simulink model "Demo2022b"  (R2022b)
settings: Solver=FixedStepAuto  StartTime=0.0  StopTime=inf  RelTol=1e-3  EnableMultiTasking=on
settings Model: ExtModeTrigDuration=2  Creator=bryantboatright  LastModifiedBy=bryantboatright
settings SolverCC: AutoInsertRateTranBlk=on
settings OptimizationCC: EnhancedBackFolding=on  PassReuseOutputArgsAs=Individual arguments  ZeroExternalMemoryAtStartup=off  ZeroInternalMemoryAtStartup=off  MaxStackSize=64  OptimizeBlockOrder=speed  DifferentSizesBufferReuse=on  OptimizationCustomize=off  EfficientTunableParamExpr=on
settings DebuggingCC: ParameterTunabilityLossMsg=error
settings HardwareCC: ProdBitPerInt=16  ProdBitPerPointer=16  ProdBitPerSizeT=16  ProdBitPerPtrDiffT=16  ProdLargestAtomicFloat=None  ProdWordSize=8  ProdHWDeviceType=Atmel->AVR
settings RTWCC: Description=Embedded Coder  SystemTargetFile=ert.tlc  HardwareBoard=Arduino Uno  TLCOptions=-aInlineSetEventsForThisBaseRateFcn=TLC_FALSE -aSuppressMultiTaskScheduler=TLC_FALSE -aRateBasedStepFcn=1  TemplateMakefile=ert_default_tmf  Toolchain=Arduino AVR  BuildConfiguration=Faster Runs
settings CodeAppCC: ForceParamTrailComments=on  IgnoreCustomStorageClasses=off  OperatorAnnotations=on  SimulinkDataObjDesc=on  SFDataObjDesc=on  InsertBlockDesc=on
settings ERTTargetCC: TargetLangStandard=C99 (ISO)  SupportContinuousTime=on  SupportVariableSizeSignals=on  ExtModeTransport=3  ExtModeStaticAlloc=on  ExtModeAutomaticAllocSize=off  ExtModeStaticAllocSize=250  ExtModeMexFile=ext_xcp  ExtModeIntrfLevel=Level2 - Open

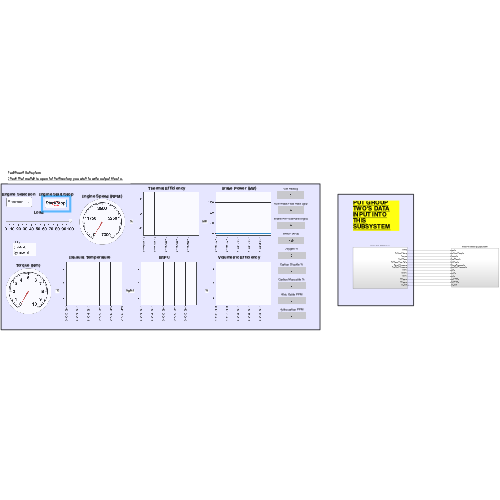
[thumbnail: Simulink's stored preview of the top-level diagram]
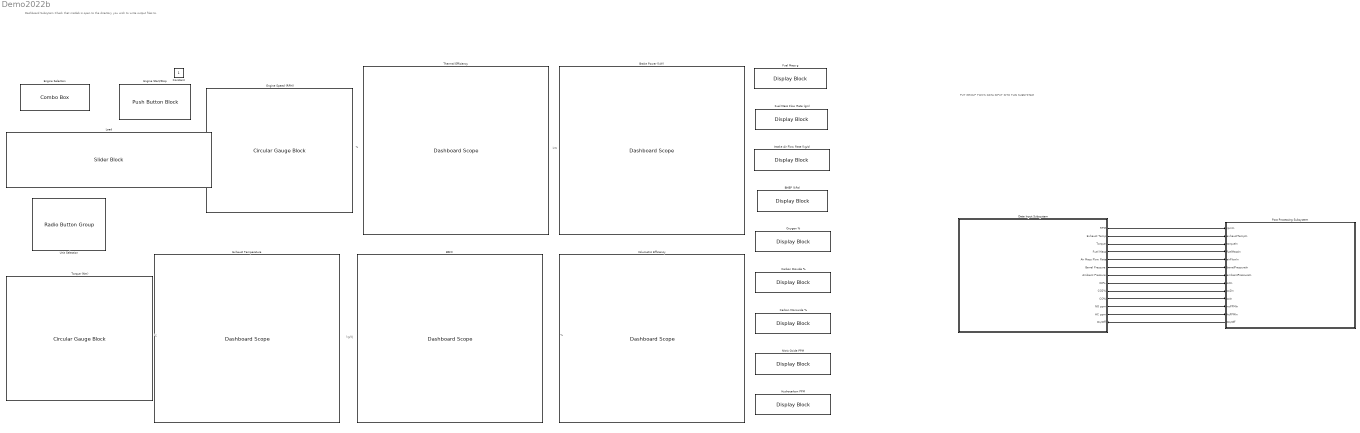
== system Demo2022b ==
  note: %
  note: Dashboard Subsytem
      |
      | Check that matlab is open to the directory you wish to write output files to.
  note: PUT GROUP TWO'S DATA INPUT INTO THIS SUBSYSTEM
  note: ˚C
  note: kg/kJ
  note: kW
  note: %
  BMEP (kPa) : DisplayBlock  LabelPosition=Hide  Transparency=1
  BSFC : DashboardScope  LegendPosition=Hide  UpdateMode=Scroll
  Brake Power (kW) : DashboardScope  LegendPosition=Hide  UpdateMode=Scroll
  Carbon Dioxide % : DisplayBlock  LabelPosition=Hide  Transparency=1
  Carbon Monoxide % : DisplayBlock  LabelPosition=Hide  Transparency=1
  Data Input Subsystem : Subsystem
      settings: PortSchema="{\"entries\":[{\"content\":{\"sides\":[{\"content\":{\"connectorIds\":[]},\"type\":\"ConnectorPlacement.EquallySpacedRectSide\",\"uuid\":\"3754a3e3-4518-42e3-a0cd-0eb816f7e60c\"},{\"content\":{\"connectorIds\":[\"Out1\",\"Out2\",\"Out3\",\"Out4\",\"Out5\",\"Out6\",\"Out7\",\"Out8\",\"Out9\",\"Out10\",\"Out11\",\"Out12\",\"In1\"],\"side\":\"RIGHT\"},\"type\":\"ConnectorPlacement.EquallySpacedRectSide\",\"uuid\":\"d3dfe676-b6e6-4c7f-98c7-8b108f201c07\"},{\"content\":{\"connectorIds\":[],\"side\":\"TOP\"},\"type\":\"ConnectorPlacement.EquallySpacedRectSide\",\"uuid\":\"2f91c8dd-0198-445b-930d-495fc8bcc849\"}]},\"type\":\"ConnectorPlacement.EquallySpacedConnector\",\"uuid\":\"520c6fba-fa44-47d2-96c9-29e04e3d0d93\"}],\"packageUris\":[\"http://schema.mathworks.com/mf0/Connector/R2020b\"],\"version\":\"1.0\"}"
  Engine Selection : ComboBox  LabelPosition=Hide  SelectedLabel=Yanmar
      settings: Values={{'Yanmar', 'Craftsman', 'John Deer', 'Chevy V6', 'Kohler', 'DuroMax'}, [1 2 3 4 5 6]}
  Engine Speed (RPM) : CircularGaugeBlock  LabelPosition=Hide  ScaleMax=7000  TickInterval=1750
  Engine Start/Stop : PushButtonBlock  ButtonText=Start/Stop  ButtonType=Latch  Icon=Engine  IconAlignment=Center  IconColor=On  OffValue=0.000000
  Exhaust Temperature : DashboardScope  LegendPosition=Hide  ScaleAtStop=off
  Fuel Mass Flow Rate (g/s) : DisplayBlock  LabelPosition=Hide  Transparency=1
  Fuel Mass g : DisplayBlock  LabelPosition=Hide  Transparency=1
  Hydrocarbon PPM : DisplayBlock  LabelPosition=Hide  Transparency=1
  Intake Air Flow Rate (kg/s) : DisplayBlock  LabelPosition=Hide  Transparency=1
  Load : SliderBlock  LabelPosition=Hide
  Nitric Oxide PPM : DisplayBlock  LabelPosition=Hide  Transparency=1
  Oxygen % : DisplayBlock  LabelPosition=Hide  Transparency=1
  Post Processing Subsystem : Subsystem
      settings: PortSchema="{\"entries\":[{\"content\":{\"sides\":[{\"content\":{\"connectorIds\":[\"In1\",\"In2\",\"In3\",\"In4\",\"In5\",\"In6\",\"In7\",\"In8\",\"In9\",\"In10\",\"In11\",\"In12\",\"Out1\"]},\"type\":\"ConnectorPlacement.EquallySpacedRectSide\",\"uuid\":\"2e8fbbbd-04f3-4cfb-b1cc-1db1e48dc879\"},{\"content\":{\"connectorIds\":[],\"side\":\"RIGHT\"},\"type\":\"ConnectorPlacement.EquallySpacedRectSide\",\"uuid\":\"1e86395c-1e99-406b-884b-92366c924b1f\"},{\"content\":{\"connectorIds\":[],\"side\":\"TOP\"},\"type\":\"ConnectorPlacement.EquallySpacedRectSide\",\"uuid\":\"23f1f2f5-9354-4dfe-ba19-9e9e16993f9b\"}]},\"type\":\"ConnectorPlacement.EquallySpacedConnector\",\"uuid\":\"bb08251b-5f96-4a99-a638-0e0833315a09\"}],\"packageUris\":[\"http://schema.mathworks.com/mf0/Connector/R2020b\"],\"version\":\"1.0\"}"
  Thermal Efficiency : DashboardScope  LegendPosition=Hide  UpdateMode=Scroll
  Torque (Nm) : CircularGaugeBlock  LabelPosition=Hide  ScaleMax=10  TickInterval=1
  Unit Selection : RadioButtonGroup  LabelPosition=Hide  SelectedLabel=Imperial  ButtonGroupName=Units
      settings: Values={{'Metric', 'Imperial'}, [0 1]}
  Volumetric Efficiency : DashboardScope  LegendPosition=Hide  UpdateMode=Scroll
  Constant : Constant  IOType=siggen
  wires:
  Data Input Subsystem/1(RPM) -> Post Processing Subsystem/1(rpmIn)
  Data Input Subsystem/2(Exhaust Temp) -> Post Processing Subsystem/2(exhaustTempIn)
  Data Input Subsystem/3(Torque) -> Post Processing Subsystem/3(torqueIn)
  Data Input Subsystem/4(Fuel Mass) -> Post Processing Subsystem/4(fuelMassIn)
  Data Input Subsystem/5(Air Mass Flow Rate) -> Post Processing Subsystem/5(airFlowIn)
  Data Input Subsystem/6(Barrel Pressure) -> Post Processing Subsystem/6(barrelPressureIn)
  Data Input Subsystem/7(Ambient Pressure) -> Post Processing Subsystem/7(ambientPressureIn)
  Data Input Subsystem/8(O2%) -> Post Processing Subsystem/8(o2In)
  Data Input Subsystem/9(CO2%) -> Post Processing Subsystem/9(co2In)
  Data Input Subsystem/10(CO%) -> Post Processing Subsystem/10(coIn)
  Data Input Subsystem/11(NO ppm) -> Post Processing Subsystem/11(noPPMIn)
  Data Input Subsystem/12(HC ppm) -> Post Processing Subsystem/12(hcPPMIn)
  Post Processing Subsystem/1(On/Off) -> Data Input Subsystem/1(On/Off)

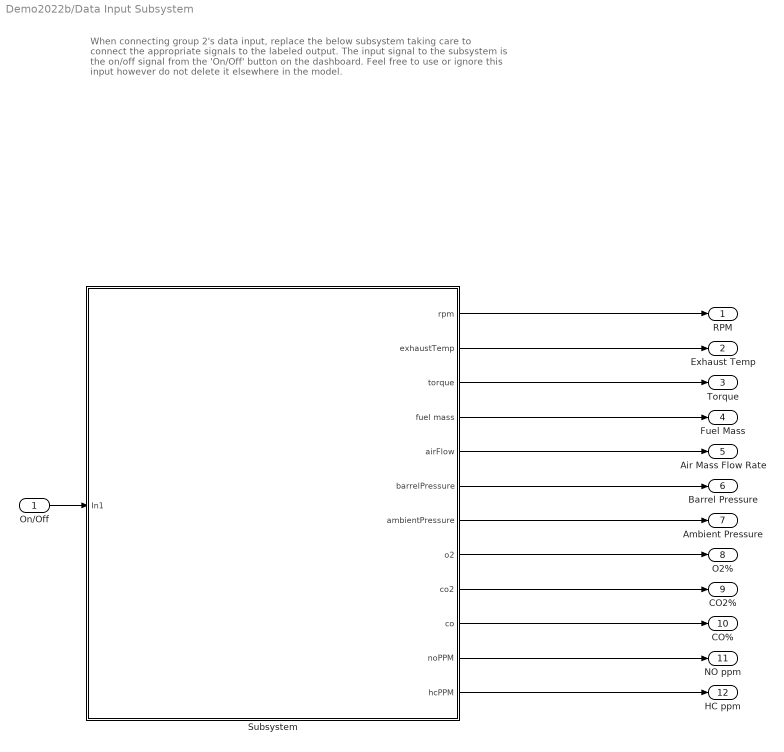
== system Demo2022b/Data Input Subsystem ==
  note: When connecting group 2's data input, replace the below subsystem taking care to connect the appropriate signals to the labeled output. The input signal to the subsystem is the on/off signal from the 'On/Off' button on the dashboard. Feel free to use or ignore this input however do not delete it elsewhere in the model.
  On/Off : Inport
  Subsystem : Subsystem
  RPM : Outport
  Exhaust Temp : Outport  Port=2
  Torque : Outport  Port=3
  Fuel Mass : Outport  Port=4
  Air Mass Flow Rate : Outport  Port=5
  Barrel Pressure : Outport  Port=6
  Ambient Pressure : Outport  Port=7
  O2% : Outport  Port=8
  CO2% : Outport  Port=9
  CO% : Outport  Port=10
  NO ppm : Outport  Port=11
  HC ppm : Outport  Port=12
  wires:
  Subsystem/1(rpm) -> RPM/1
  Subsystem/2(exhaustTemp) -> Exhaust Temp/1
  Subsystem/3(torque) -> Torque/1
  Subsystem/4(fuel mass) -> Fuel Mass/1
  Subsystem/5(airFlow) -> Air Mass Flow Rate/1
  Subsystem/6(barrelPressure) -> Barrel Pressure/1
  Subsystem/7(ambientPressure) -> Ambient Pressure/1
  Subsystem/8(o2) -> O2%/1
  Subsystem/9(co2) -> CO2%/1
  Subsystem/10(co) -> CO%/1
  Subsystem/11(noPPM) -> NO ppm/1
  Subsystem/12(hcPPM) -> HC ppm/1
  On/Off/1 -> Subsystem/1(In1)

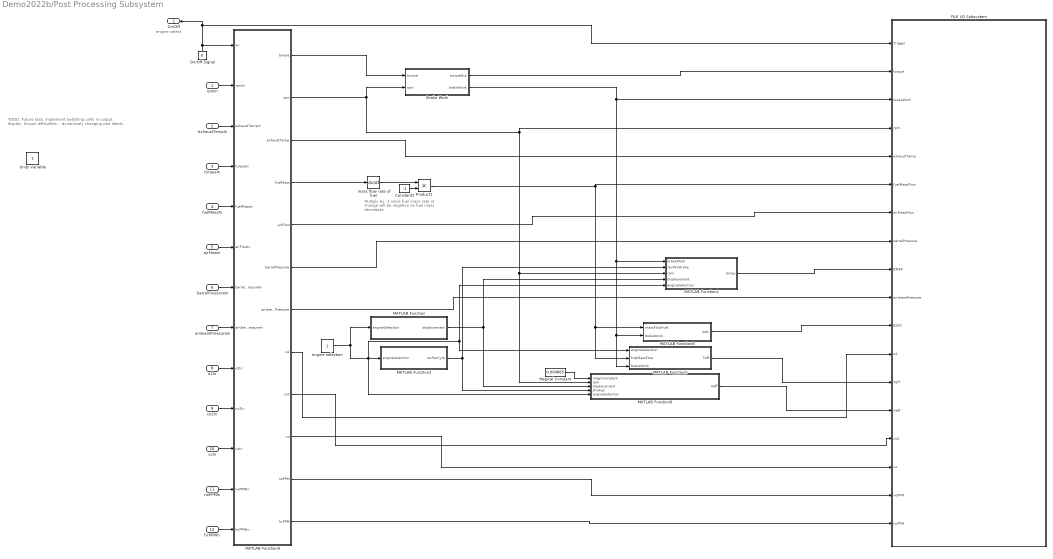
== system Demo2022b/Post Processing Subsystem ==
  note: Multiply by -1 since fuel mass rate of
      | change will be negative as fuel mass
      | decreases.
  note: TODO: Future task, implement switching units in output display.
      |
      | Known difficulties:
      | - dynamicaly changing plot labels.
  note: engine select
  rpmIn : Inport
  exhaustTempIn : Inport  Port=2
  torqueIn : Inport  Port=3
  fuelMassIn : Inport  Port=4
  airFlowIn : Inport  Port=5
  barrelPressureIn : Inport  Port=6
  ambientPressureIn : Inport  Port=7
  o2In : Inport  Port=8
  co2In : Inport  Port=9
  coIn : Inport  Port=10
  noPPMIn : Inport  Port=11
  hcPPMIn : Inport  Port=12
  Brake Work : MATLAB Function  TreatAsAtomicUnit=on
  Constant2 : Constant  Value=-1
  FILE I/O Subsystem : Subsystem
  MATLAB Function : MATLAB Function  TreatAsAtomicUnit=on
  MATLAB Function1 : MATLAB Function  TreatAsAtomicUnit=on
  MATLAB Function2 : MATLAB Function  TreatAsAtomicUnit=on
  MATLAB Function5 : MATLAB Function  TreatAsAtomicUnit=on
  MATLAB Function6 : MATLAB Function  TreatAsAtomicUnit=on
  MATLAB Function8 : MATLAB Function  TreatAsAtomicUnit=on
  MATLAB Function9 : MATLAB Function  TreatAsAtomicUnit=on
  Magical Constant : Constant  Value=0.004865
  On/Off Signal : Constant  Value=0
  Product1 : Product
  Units Variable : Constant
  engine selection : Constant
  mass flow rate of fuel : Derivative
  On/Off : Outport
  wires:
  Brake Work/2(brakeWork) -> MATLAB Function5/3(brakeWork), MATLAB Function8/2(brakeWork), MATLAB Function1/1(brakeWork), FILE I/O Subsystem/3(brakeWork)
  MATLAB Function2/1(revPerCyle) -> MATLAB Function1/2(revPerStroke), MATLAB Function6/4(strokes)
  Magical Constant/1 -> MATLAB Function6/1(magicConstant)
  MATLAB Function/1(displacement) -> MATLAB Function1/4(displacement), MATLAB Function6/3(displacement)
  hcPPMIn/1 -> MATLAB Function9/13(hcPPMIn)
  MATLAB Function9/4(fuelMass) -> mass flow rate of fuel/1
  MATLAB Function9/2(rpm) -> Brake Work/2(rpm), MATLAB Function6/2(rpm), MATLAB Function1/3(rpm), FILE I/O Subsystem/4(rpm)
  noPPMIn/1 -> MATLAB Function9/12(noPPMIn)
  MATLAB Function9/1(torque) -> Brake Work/1(torque)
  coIn/1 -> MATLAB Function9/11(coIn)
  engine selection/1 -> MATLAB Function/1(engineSelection), MATLAB Function6/5(engineSelection), MATLAB Function1/5(engineSelection), MATLAB Function5/1(engineSelection), MATLAB Function2/1(engineSelection)
  co2In/1 -> MATLAB Function9/10(co2In)
  exhaustTempIn/1 -> MATLAB Function9/3(exhaustTempIn)
  ambientPressureIn/1 -> MATLAB Function9/8(ambientPressureIn)
  rpmIn/1 -> MATLAB Function9/2(rpmIn)
  fuelMassIn/1 -> MATLAB Function9/5(fuelMassIn)
  o2In/1 -> MATLAB Function9/9(o2In)
  barrelPressureIn/1 -> MATLAB Function9/7(barrelPressureIn)
  torqueIn/1 -> MATLAB Function9/4(torqueIn)
  airFlowIn/1 -> MATLAB Function9/6(airFlowIn)
  On/Off Signal/1 -> On/Off/1, FILE I/O Subsystem/1(Trigger), MATLAB Function9/1(on)
  Constant2/1 -> Product1/2
  Product1/1 -> MATLAB Function5/2(fuelMassFlow), MATLAB Function8/1(massFlowFuel), FILE I/O Subsystem/6(fuelMassFlow)
  mass flow rate of fuel/1 -> Product1/1
  Brake Work/1(torqueOut) -> FILE I/O Subsystem/2(torque)
  MATLAB Function9/3(exhaustTemp) -> FILE I/O Subsystem/5(exhaustTemp)
  MATLAB Function9/5(airFlow) -> FILE I/O Subsystem/7(airMassFlow)
  MATLAB Function9/6(barrelPressure) -> FILE I/O Subsystem/8(barrelPressure)
  MATLAB Function1/1(bmep) -> FILE I/O Subsystem/9(BMEP)
  MATLAB Function9/7(ambientPressure) -> FILE I/O Subsystem/10(ambientPressure)
  MATLAB Function8/1(bsfc) -> FILE I/O Subsystem/11(BSFC)
  MATLAB Function9/8(o2) -> FILE I/O Subsystem/12(o2)
  MATLAB Function5/1(Teff) -> FILE I/O Subsystem/13(Teff)
  MATLAB Function6/1(Veff) -> FILE I/O Subsystem/14(Veff)
  MATLAB Function9/9(co2) -> FILE I/O Subsystem/15(co2)
  MATLAB Function9/10(co) -> FILE I/O Subsystem/16(co)
  MATLAB Function9/11(noPPM) -> FILE I/O Subsystem/17(noPPM)
  MATLAB Function9/12(hcPPM) -> FILE I/O Subsystem/18(hcPPM)

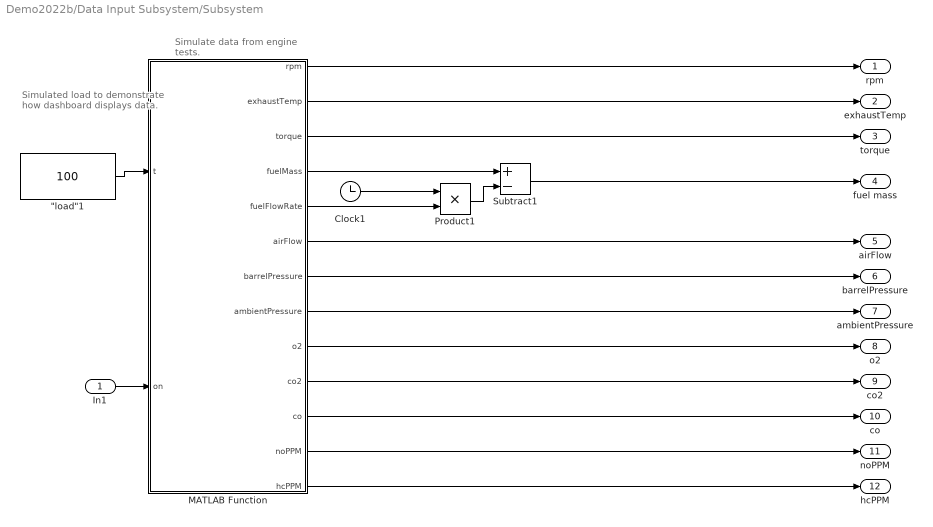
== system Demo2022b/Data Input Subsystem/Subsystem ==
  note: Simulated load to demonstrate how
      | dashboard displays data.
  note: Simulate data from engine
      | tests.
  In1 : Inport
  "\"load\"1" : Constant  Value=100
  Clock1 : Clock
  MATLAB Function : MATLAB Function  TreatAsAtomicUnit=on
  Product1 : Product
  Subtract1 : Sum  Inputs=+-
  rpm : Outport
  exhaustTemp : Outport  Port=2
  torque : Outport  Port=3
  fuel mass : Outport  Port=4
  airFlow : Outport  Port=5
  barrelPressure : Outport  Port=6
  ambientPressure : Outport  Port=7
  o2 : Outport  Port=8
  co2 : Outport  Port=9
  co : Outport  Port=10
  noPPM : Outport  Port=11
  hcPPM : Outport  Port=12
  wires:
  MATLAB Function/3(torque) -> torque/1
  MATLAB Function/13(hcPPM) -> hcPPM/1
  MATLAB Function/6(airFlow) -> airFlow/1
  MATLAB Function/5(fuelFlowRate) -> Product1/2
  MATLAB Function/12(noPPM) -> noPPM/1
  MATLAB Function/7(barrelPressure) -> barrelPressure/1
  MATLAB Function/8(ambientPressure) -> ambientPressure/1
  In1/1 -> MATLAB Function/2(on)
  MATLAB Function/9(o2) -> o2/1
  "\"load\"1"/1 -> MATLAB Function/1(t)
  MATLAB Function/4(fuelMass) -> Subtract1/1
  MATLAB Function/11(co) -> co/1
  MATLAB Function/10(co2) -> co2/1
  Product1/1 -> Subtract1/2
  Clock1/1 -> Product1/1
  Subtract1/1 -> fuel mass/1
  MATLAB Function/2(exhaustTemp) -> exhaustTemp/1
  MATLAB Function/1(rpm) -> rpm/1

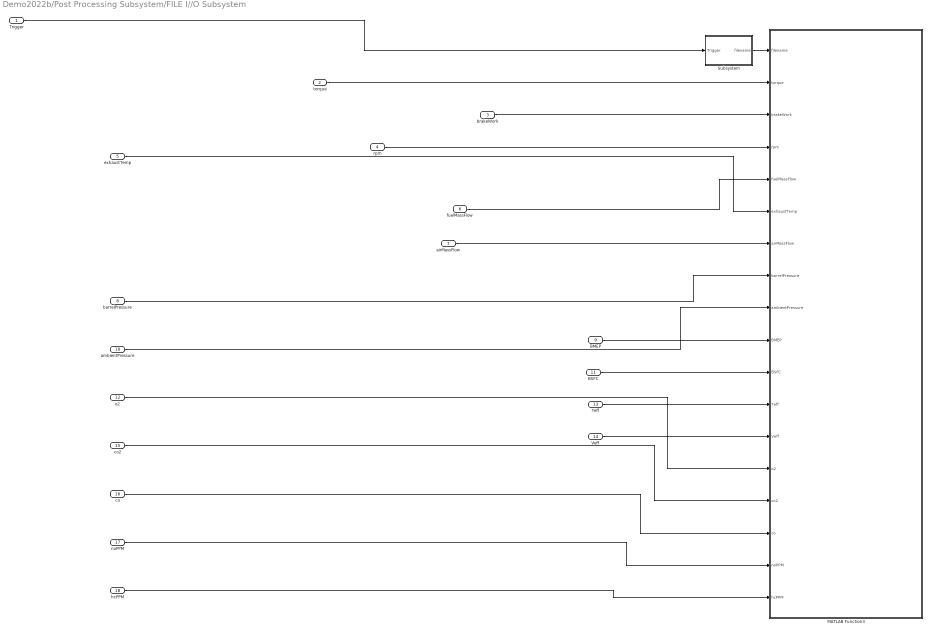
== system Demo2022b/Post Processing Subsystem/FILE I//O Subsystem ==
  Trigger : Inport
  torque : Inport  Port=2
  brakeWork : Inport  Port=3
  rpm : Inport  Port=4
  exhaustTemp : Inport  Port=5
  fuelMassFlow : Inport  Port=6
  airMassFlow : Inport  Port=7
  barrelPressure : Inport  Port=8
  BMEP : Inport  Port=9
  ambientPressure : Inport  Port=10
  BSFC : Inport  Port=11
  o2 : Inport  Port=12
  Teff : Inport  Port=13
  Veff : Inport  Port=14
  co2 : Inport  Port=15
  co : Inport  Port=16
  noPPM : Inport  Port=17
  hcPPM : Inport  Port=18
  MATLAB Function3 : MATLAB Function  TreatAsAtomicUnit=on
  Subsystem : Subsystem
  wires:
  noPPM/1 -> MATLAB Function3/17(noPPM)
  brakeWork/1 -> MATLAB Function3/3(brakeWork)
  exhaustTemp/1 -> MATLAB Function3/6(exhaustTemp)
  Veff/1 -> MATLAB Function3/13(Veff)
  barrelPressure/1 -> MATLAB Function3/8(barrelPressure)
  fuelMassFlow/1 -> MATLAB Function3/5(fuelMassFlow)
  o2/1 -> MATLAB Function3/14(o2)
  torque/1 -> MATLAB Function3/2(torque)
  Trigger/1 -> Subsystem/1(Trigger)
  Teff/1 -> MATLAB Function3/12(Teff)
  ambientPressure/1 -> MATLAB Function3/9(ambientPressure)
  BMEP/1 -> MATLAB Function3/10(BMEP)
  hcPPM/1 -> MATLAB Function3/18(hcPPM)
  airMassFlow/1 -> MATLAB Function3/7(airMassFlow)
  co/1 -> MATLAB Function3/16(co)
  Subsystem/1(filename) -> MATLAB Function3/1(filename)
  rpm/1 -> MATLAB Function3/4(rpm)
  co2/1 -> MATLAB Function3/15(co2)
  BSFC/1 -> MATLAB Function3/11(BSFC)

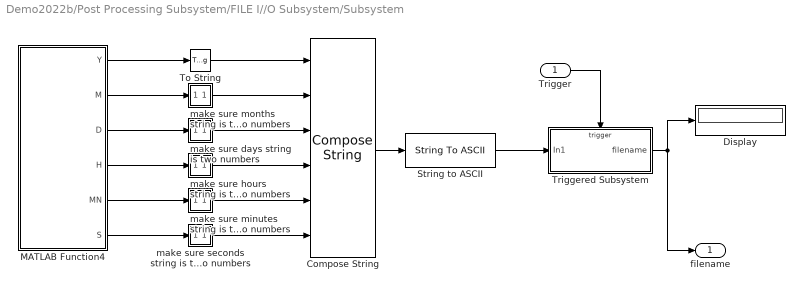
== system Demo2022b/Post Processing Subsystem/FILE I//O Subsystem/Subsystem ==
  Trigger : Inport
  Compose String : ComposeString  Format="\"%s-%s-%s--%s-%s-%s-output.csv\""
  Display : Display
  MATLAB Function4 : MATLAB Function  TreatAsAtomicUnit=on  SystemSampleTime=200
  String to ASCII : StringToASCII
  To String : ToString
  Triggered Subsystem : Subsystem  TreatAsAtomicUnit=on
  make sure days string is two numbers : Subsystem
  make sure hours string is two numbers : Subsystem
  make sure minutes string is two numbers : Subsystem
  make sure months string is two numbers : Subsystem
  make sure seconds string is two numbers : Subsystem
  filename : Outport
  wires:
  make sure months string is two numbers/1(Out1) -> Compose String/2
  To String/1 -> Compose String/1
  MATLAB Function4/6(S) -> make sure seconds string is two numbers/1(In1)
  Compose String/1 -> String to ASCII/1
  MATLAB Function4/5(MN) -> make sure minutes string is two numbers/1(In1)
  make sure days string is two numbers/1(Out1) -> Compose String/3
  make sure minutes string is two numbers/1(Out1) -> Compose String/5
  MATLAB Function4/4(H) -> make sure hours string is two numbers/1(In1)
  make sure hours string is two numbers/1(Out1) -> Compose String/4
  Trigger/1 -> Triggered Subsystem/Trigger
  MATLAB Function4/2(M) -> make sure months string is two numbers/1(In1)
  Triggered Subsystem/1(filename) -> filename/1, Display/1
  MATLAB Function4/3(D) -> make sure days string is two numbers/1(In1)
  MATLAB Function4/1(Y) -> To String/1
  make sure seconds string is two numbers/1(Out1) -> Compose String/6
  String to ASCII/1 -> Triggered Subsystem/1(In1)

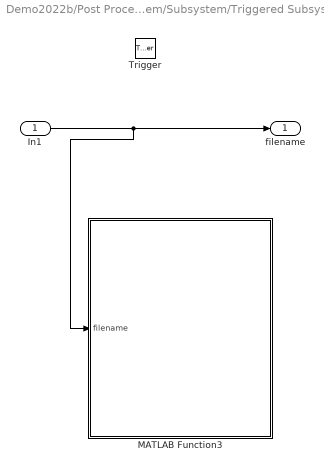
== system Demo2022b/Post Processing Subsystem/FILE I//O Subsystem/Subsystem/Triggered Subsystem ==
  In1 : Inport
  Trigger : TriggerPort  VariantControl=(inherit)
  MATLAB Function3 : MATLAB Function  TreatAsAtomicUnit=on
  filename : Outport
  wires:
  In1/1 -> MATLAB Function3/1(filename), filename/1

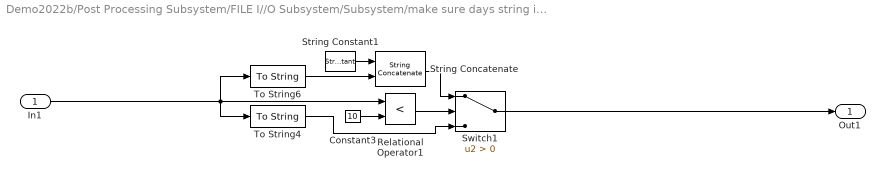
== system Demo2022b/Post Processing Subsystem/FILE I//O Subsystem/Subsystem/make sure days string is two numbers ==
  In1 : Inport
  Constant3 : Constant  Value=10  VectorParams1D=off  OutDataTypeStr=int8
  Relational Operator1 : RelationalOperator  Operator=<  OutDataTypeStr=boolean  RndMeth=Simplest  InputSameDT=off
  String Concatenate : StringConcatenate
  String Constant1 : StringConstant  String="\"0\""
  Switch1 : Switch  Criteria=u2 > Threshold  SaturateOnIntegerOverflow=off  InputSameDT=off
  To String4 : ToString
  To String6 : ToString
  Out1 : Outport
  wires:
  Constant3/1 -> Relational Operator1/2
  Relational Operator1/1 -> Switch1/2
  To String4/1 -> Switch1/3
  To String6/1 -> String Concatenate/2
  String Constant1/1 -> String Concatenate/1
  String Concatenate/1 -> Switch1/1
  In1/1 -> Relational Operator1/1, To String4/1, To String6/1
  Switch1/1 -> Out1/1

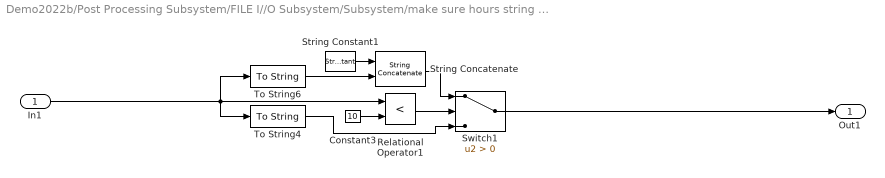
== system Demo2022b/Post Processing Subsystem/FILE I//O Subsystem/Subsystem/make sure hours string is two numbers ==
  In1 : Inport
  Constant3 : Constant  Value=10  VectorParams1D=off  OutDataTypeStr=int8
  Relational Operator1 : RelationalOperator  Operator=<  OutDataTypeStr=boolean  RndMeth=Simplest  InputSameDT=off
  String Concatenate : StringConcatenate
  String Constant1 : StringConstant  String="\"0\""
  Switch1 : Switch  Criteria=u2 > Threshold  SaturateOnIntegerOverflow=off  InputSameDT=off
  To String4 : ToString
  To String6 : ToString
  Out1 : Outport
  wires:
  Switch1/1 -> Out1/1
  In1/1 -> To String6/1, To String4/1, Relational Operator1/1
  String Concatenate/1 -> Switch1/1
  String Constant1/1 -> String Concatenate/1
  To String6/1 -> String Concatenate/2
  To String4/1 -> Switch1/3
  Relational Operator1/1 -> Switch1/2
  Constant3/1 -> Relational Operator1/2

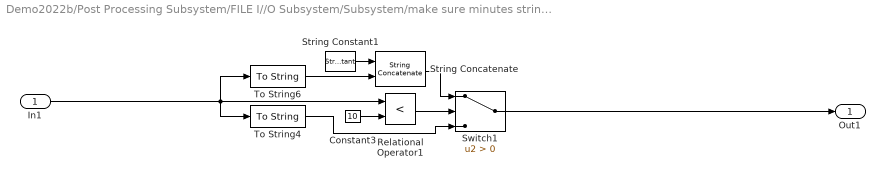
== system Demo2022b/Post Processing Subsystem/FILE I//O Subsystem/Subsystem/make sure minutes string is two numbers ==
  In1 : Inport
  Constant3 : Constant  Value=10  VectorParams1D=off  OutDataTypeStr=int8
  Relational Operator1 : RelationalOperator  Operator=<  OutDataTypeStr=boolean  RndMeth=Simplest  InputSameDT=off
  String Concatenate : StringConcatenate
  String Constant1 : StringConstant  String="\"0\""
  Switch1 : Switch  Criteria=u2 > Threshold  SaturateOnIntegerOverflow=off  InputSameDT=off
  To String4 : ToString
  To String6 : ToString
  Out1 : Outport
  wires:
  Constant3/1 -> Relational Operator1/2
  Relational Operator1/1 -> Switch1/2
  To String4/1 -> Switch1/3
  To String6/1 -> String Concatenate/2
  String Constant1/1 -> String Concatenate/1
  String Concatenate/1 -> Switch1/1
  In1/1 -> Relational Operator1/1, To String4/1, To String6/1
  Switch1/1 -> Out1/1

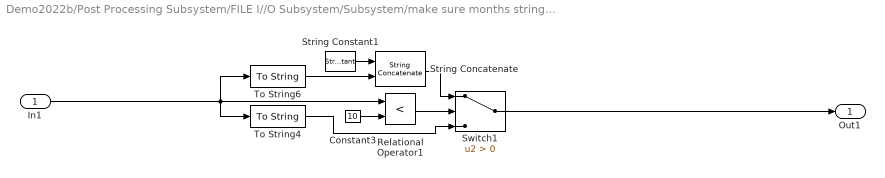
== system Demo2022b/Post Processing Subsystem/FILE I//O Subsystem/Subsystem/make sure months string is two numbers ==
  In1 : Inport
  Constant3 : Constant  Value=10  VectorParams1D=off  OutDataTypeStr=int8
  Relational Operator1 : RelationalOperator  Operator=<  OutDataTypeStr=boolean  RndMeth=Simplest  InputSameDT=off
  String Concatenate : StringConcatenate
  String Constant1 : StringConstant  String="\"0\""
  Switch1 : Switch  Criteria=u2 > Threshold  SaturateOnIntegerOverflow=off  InputSameDT=off
  To String4 : ToString
  To String6 : ToString
  Out1 : Outport
  wires:
  Switch1/1 -> Out1/1
  In1/1 -> To String6/1, To String4/1, Relational Operator1/1
  String Concatenate/1 -> Switch1/1
  String Constant1/1 -> String Concatenate/1
  To String6/1 -> String Concatenate/2
  To String4/1 -> Switch1/3
  Relational Operator1/1 -> Switch1/2
  Constant3/1 -> Relational Operator1/2

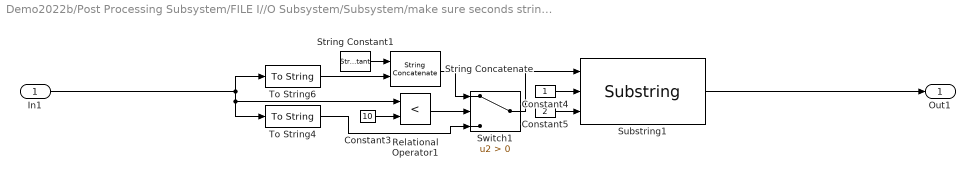
== system Demo2022b/Post Processing Subsystem/FILE I//O Subsystem/Subsystem/make sure seconds string is two numbers ==
  In1 : Inport
  Constant3 : Constant  Value=10  VectorParams1D=off  OutDataTypeStr=int8
  Constant4 : Constant  VectorParams1D=off  OutDataTypeStr=int8
  Constant5 : Constant  Value=2  VectorParams1D=off  OutDataTypeStr=uint8
  Relational Operator1 : RelationalOperator  Operator=<  OutDataTypeStr=boolean  RndMeth=Simplest  InputSameDT=off
  String Concatenate : StringConcatenate
  String Constant1 : StringConstant  String="\"0\""
  Substring1 : Substring
  Switch1 : Switch  Criteria=u2 > Threshold  SaturateOnIntegerOverflow=off  InputSameDT=off
  To String4 : ToString
  To String6 : ToString
  Out1 : Outport
  wires:
  Substring1/1 -> Out1/1
  To String4/1 -> Switch1/3
  Switch1/1 -> Substring1/1
  Constant3/1 -> Relational Operator1/2
  Constant5/1 -> Substring1/3
  In1/1 -> Relational Operator1/1, To String4/1, To String6/1
  Constant4/1 -> Substring1/2
  Relational Operator1/1 -> Switch1/2
  To String6/1 -> String Concatenate/2
  String Constant1/1 -> String Concatenate/1
  String Concatenate/1 -> Switch1/1

== matlab function Demo2022b/Post Processing Subsystem/MATLAB Function6 ==
  data: magicConstant input; Veff output; rpm input; displacement input; strokes input; engineSelection input
% Calculate Volumetric Efficiency
function Veff = calcVolumetricEfficiency(magicConstant, rpm, displacement, strokes, engineSelection)
if(engineSelection == 1 || engineSelection == 2 || engineSelection == 5 || engineSelection == 6)
    Veff = ((strokes * magicConstant) / (1.205 * displacement * (rpm / 60)));
elseif (engineSelection == 3)
    Veff = ((strokes * magicConstant) / (1.205 * (displacement * 4) * (rpm / 60)));
else
    Veff = ((strokes * magicConstant) / (1.205 * (displacement * 6) * (rpm / 60)));
end

== matlab function Demo2022b/Post Processing Subsystem/FILE I//O Subsystem/Subsystem/MATLAB Function4 ==
  data: Y output; M output; D output; H output; MN output; S output
function [Y, M, D, H, MN, S] = dateGenerator()
   Y = 0;
   M = 0;
   D = 0;
   H = 0;
   MN = 0;
   S = 0;
   [Y, M, D, H, MN, S] = datevec(datetime("now"));
end

== matlab function Demo2022b/Post Processing Subsystem/MATLAB Function8 ==
  data: massFlowFuel input; bsfc output; brakeWork input
% calculate BSFC based on fuel mass flow rate (kg/s) and Brake Work (Nm).
function bsfc = calcBSFC(massFlowFuel,brakeWork)

bsfc = massFlowFuel./brakeWork;

== matlab function Demo2022b/Post Processing Subsystem/MATLAB Function9 ==
  data: torque output; rpm output; exhaustTemp output; fuelMass output; airFlow output; barrelPressure output; ambientPressure output; on input; o2 output; co2 output; co output; noPPM output; hcPPM output; rpmIn input; exhaustTempIn input; torqueIn input; fuelMassIn input; airFlowIn input; barrelPressureIn input; ambientPressureIn input; o2In input; co2In input; coIn input; noPPMIn input; hcPPMIn input
% function to take input of 
%
% returns:
%
%   rpm: engine     speed rev per minute
%   exhaustTemp:    exhaust temperature in celsius
%   torque:         torque in Newton-meters
%   torqueMeasured: boolean - true if torque is measured, false if not
%   volts:          voltage
%   amps:           current
%   fuelMass:       mass of fuel container at current time.
%   

function [ torque,rpm,exhaustTemp,fuelMass,airFlow,barrelPressure,ambientPressure,...
    o2,co2,co,noPPM,hcPPM ] = fcn(on,rpmIn,exhaustTempIn,torqueIn,fuelMassIn,...
    airFlowIn,barrelPressureIn,ambientPressureIn,o2In,co2In,coIn,noPPMIn,hcPPMIn)
if(on == 1)
    rpm = rpmIn;
    exhaustTemp = exhaustTempIn;
    torque = torqueIn;
    fuelMass = fuelMassIn;
    airFlow = airFlowIn;
    barrelPressure = barrelPressureIn;
    ambientPressure = ambientPressureIn;
    o2 = o2In;
    co2 = co2In;
    co = coIn;
    noPPM = noPPMIn;
    hcPPM = hcPPMIn;
else
    rpm = 0;
    exhaustTemp = 0;
    torque = 0;
    fuelMass = 0;
    airFlow = 0;
    barrelPressure = 0;
    ambientPressure = 0;
    o2 = 0;
    co2 = 0;
    co = 0;
    noPPM = 0;
    hcPPM = 0;
end

== matlab function Demo2022b/Post Processing Subsystem/FILE I//O Subsystem/MATLAB Function3 ==
  data: filename input; torque input; brakeWork input; rpm input; fuelMassFlow input; exhaustTemp input; airMassFlow input; barrelPressure input; ambientPressure input; BMEP input; BSFC input; Teff input; Veff input; o2 input; co2 input; co input; noPPM input; hcPPM input
% log file generation - currently overwrites each run
% \r\n used for windows line termination style CRLF - switch to just \n if
% using unix like system
function fileOutput(filename,torque,brakeWork,rpm,fuelMassFlow,exhaustTemp,airMassFlow,barrelPressure,ambientPressure,BMEP,BSFC,Teff,Veff,o2,co2,co,noPPM,hcPPM)
if ([0 0] ~= size(double(char(filename))))
    file = fopen(char(filename),'a');
    if (0 > file)
        return
    end

    fprintf(file,'%.3f,%.3f,%.3f,%.3f,%.3f,%.3f,%.3f,%.3f,%.3f,%.3f,%.3f,%.3f,%.3f,%.3f,%.3f,%.3f,%.3f\r\n', ...
        torque,brakeWork,rpm,fuelMassFlow,exhaustTemp,airMassFlow,barrelPressure,ambientPressure,BMEP,BSFC,Teff,Veff,o2,co2,co,noPPM,hcPPM);
    fclose(file);
end

== matlab function Demo2022b/Post Processing Subsystem/FILE I//O Subsystem/Subsystem/Triggered Subsystem/MATLAB Function3 ==
  data: filename input
% log file generation - currently overwrites each run
% \r\n used for windows line termination style CRLF - switch to just \n if
% using unix like system
function fileOutput(filename)

if (0 ~= size(double(char(filename))))
    file = fopen(char(filename),'a');
    if (0 > file)
        return
    end

    fprintf(file,['torque,brakeWork,rpm,fuel mass flow,exhaust temperature,air mass flow..' ...
        ',barrel pressure,ambient pressure,BMEP,BSFC,thermal efficiency,...' ...
        'volumetric efficiency,o2,co2,co,no PPM,hc PPM\r\n']);
    fclose(file);
end

== matlab function Demo2022b/Post Processing Subsystem/MATLAB Function1 ==
  data: brakeWork input; bmep output; revPerStroke input; rpm input; displacement input; engineSelection input
% Calculate Brake Mean Effective Pressure (kPa).
function bmep = calcBMEP(brakeWork, revPerStroke, rpm,  displacement, engineSelection)
if(engineSelection == 1 || engineSelection == 2 || engineSelection == 5 || engineSelection ==6)
    bmep = ((brakeWork/((rpm/60)/revPerStroke))/displacement)/1000;
elseif(engineSelection==3)
     bmep = ((brakeWork/((rpm/60)/revPerStroke))/(displacement*4))/1000;
else
     bmep = ((brakeWork/((rpm/60)/revPerStroke))/(displacement*6))/1000;
end

== matlab function Demo2022b/Post Processing Subsystem/MATLAB Function ==
  data: displacement output; engineSelection input
% Set engine displacement (m^3) based on dropdown menu choice from dashboard
function displacement = pickDisplacement(engineSelection)
data = [0.000296 0.000196 0.000475 000.0004667 0.000429 0.000225];

displacement = data(1,engineSelection);

== matlab function Demo2022b/Post Processing Subsystem/MATLAB Function2 ==
  data: revPerCyle output; engineSelection input
% Set revolutions per cycle ( 1 for 2-stroke, 2 for 4-stroke ) based on
% engine selection from drop down menu on dashboard.
function revPerCyle = pickRevPerStroke(engineSelection)
data = [4 4 4 4 4 4];
revPerCyle = data(1,engineSelection);

== matlab function Demo2022b/Post Processing Subsystem/Brake Work ==
  data: torque input; torqueOut output; rpm input; brakeWork output
% Calculate Brake Work (kW/s) based on Engine Speed (rpm) and Torque (Nm)
function [torqueOut,brakeWork] = calcBrakeWork(torque,rpm)
brakeWork = 2 * pi * (rpm/60.0) * torque;

% Using diff name to reduce confusions. Torque only used in this function
% so to clean up lines was brought into this function.
torqueOut = torque;

== matlab function Demo2022b/Data Input Subsystem/Subsystem/MATLAB Function ==
  data: t input; rpm output; on input; exhaustTemp output; torque output; fuelMass output; fuelFlowRate output; airFlow output; barrelPressure output; ambientPressure output; o2 output; co2 output; co output; noPPM output; hcPPM output
function [ rpm,exhaustTemp,torque,fuelMass,fuelFlowRate,airFlow,barrelPressure,ambientPressure,...
    o2,co2,co,noPPM,hcPPM ] = fcn(t,on)
if (on)
    data = (1 + t / 100.0) * [ 2000 125 2.258 2000.0 0.004 0.94 3.4 16.5 0.003 35 59 0.004 ];
    rpm = data(1);
    exhaustTemp = data(2);
    torque = data(3);
    fuelMass = data(4);
    airFlow = data(5);
    barrelPressure = data(6);
    ambientPressure = 29;
    o2 = data(7);
    co2 = data(8);
    co = data(9);
    noPPM = data(10);
    hcPPM = data(11);
    fuelFlowRate = data(12);
else
    rpm = 0;
    exhaustTemp = 0;
    torque = 0;
    fuelMass = 0;
    airFlow = 0;
    barrelPressure = 0;
    ambientPressure = 0;
    o2 = 0;
    co2 = 0;
    co = 0;
    noPPM = 0;
    hcPPM = 0;
    fuelFlowRate = 0;
end

== matlab function Demo2022b/Post Processing Subsystem/MATLAB Function5 ==
  data: Teff output; engineSelection input; fuelMassFlow input; brakeWork input

function Teff = calcThermalEfficiency(engineSelection, fuelMassFlow, brakeWork)

% Set lower heating value of fuel (J/kg) based on engine selection. 
lowerHeatingValues = [47.3e6 44.4e6];
Qlhv = 0;
if(engineSelection == 3)
    Qlhv = fuelMassFlow * lowerHeatingValues(1, 2);
else
    Qlhv = fuelMassFlow * lowerHeatingValues(1,1);
end

Teff = (brakeWork/Qlhv) * 100;
